simulink model "DigitalControl"  (R2015a)
settings: Solver=ode45  StartTime=0.0  StopTime=10.0  MaxStep=0.1  RelTol=1e-3
undefined symbols (not defined in the file): deltat, deltat1, fden, fnum, Ka, Kf, Ki, Kq, Tal, Ts, W1, W2
libraries: simulink x1
settings Model: FPTRunName=Active  ModifiedByFormat=The MathWorks Inc.  CovSFcnEnable=off  Creator=The MathWorks Inc.  LastModifiedBy=The MathWorks Inc.
settings ConfigSet: ConfigType=Model
settings SolverCC: Priority=auto
settings DataIOCC: SaveOutput=off  SaveTime=off  SignalLoggingName=DigitalControl
settings OptimizationCC: InlineParamsCompatibleMode=off  ExpressionDepthLimit=2147483647  InitFltsAndDblsToZero=on  ForceBlockIOInitOptimize=off  EvaledLifeSpan=1  SimCompilerOptimization=Off
settings DebuggingCC: SaveWithParameterizedLinksMsg=none  UnderspecifiedInitializationDetection=Classic  MergeDetectMultiDrivingBlocksExec=none  SignalResolutionControl=TryResolveAllWithWarning  SolverPrmCheckMsg=warning  MultiTaskDSMMsg=warning  MultiTaskCondExecSysMsg=none  FcnCallInpInsideContextMsg=UseLocalSettings  AllowSymbolicDim=off  StateNameClashWarn=warning  SFMismatchInSimAndRtwBecauseOfMissingDataTypeDiag=warning
settings ModelReferenceCC: ModelReferenceMinAlgLoopOccurrences=on
settings RTWCC: EnableTagging=off  RTWCompilerOptimization=Off
settings CodeAppCC: ParameterTuningSideEffectCode=Output function  AllmanStyle=off
settings GRTTargetCC: TargetFcnLib=ansi_tfl_tmw.mat  CombineOutputUpdateFcns=off  EnableShiftOperators=off  PortableWordSizesTransition=off  GenerateErtSFunctionTransition=off  CreateSILPILBlockTransition=None  CodeProfilingSaveOptionsTransition=SummaryOnly  CodeExecutionProfilingTransition=off  CodeProfilingInstrumentationTransition=off  CodeExecutionProfileVariableTransition=executionProfile  GRTInterface=on

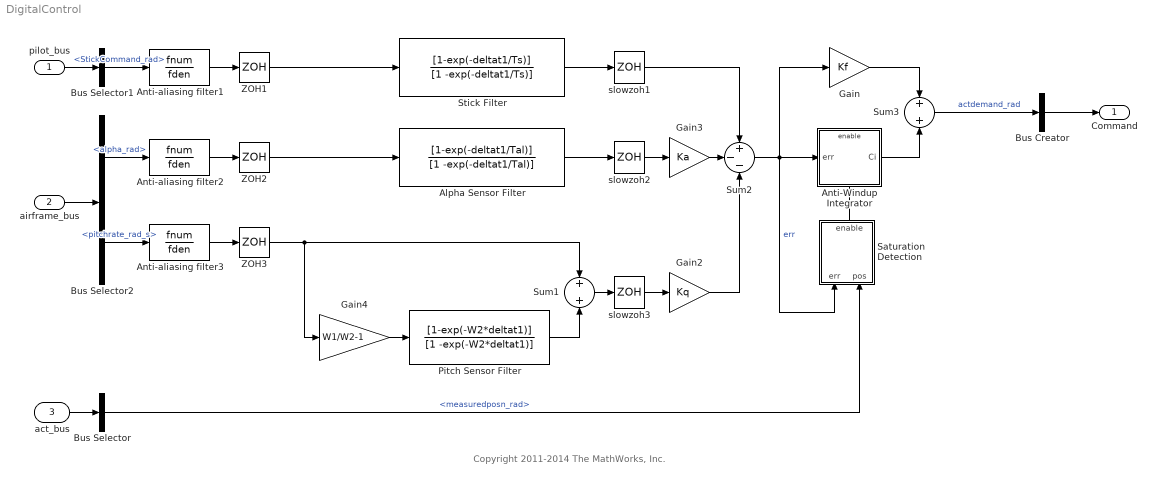
== system DigitalControl ==
  note: Copyright 2011-2014 The MathWorks, Inc.
  pilot_bus : Inport  IOType=none  Commented=off  StatePerturbationForJacobian=1.0e-05  OutDataTypeStr=Bus: PILOT_BUS
  airframe_bus : Inport  IOType=none  Commented=off  StatePerturbationForJacobian=1.0e-05  Port=2  OutDataTypeStr=Bus: AIRFRAME_BUS
  act_bus : Inport  IOType=none  Commented=off  StatePerturbationForJacobian=1.0e-05  Port=3  OutDataTypeStr=Bus: ACT_BUS
  Alpha Sensor Filter : DiscreteTransferFcn  IOType=none  Commented=off  StatePerturbationForJacobian=1.0e-05  Numerator=[1-exp(-deltat1/Tal)]  Denominator=[1 -exp(-deltat1/Tal)]  SampleTime=deltat1
  Anti-Windup Integrator : Subsystem  IOType=none  Commented=off  StatePerturbationForJacobian=1.0e-05  TreatAsAtomicUnit=on
      settings: RTWSystemCode=Inline
  Anti-aliasing filter1 : TransferFcn  IOType=none  Commented=off  StatePerturbationForJacobian=1.0e-05  Numerator=fnum  Denominator=fden
      settings: AttributesFormatString=%<Description>
  Anti-aliasing filter2 : TransferFcn  IOType=none  Commented=off  StatePerturbationForJacobian=1.0e-05  Numerator=fnum  Denominator=fden
      settings: AttributesFormatString=%<Description>
  Anti-aliasing filter3 : TransferFcn  IOType=none  Commented=off  StatePerturbationForJacobian=1.0e-05  Numerator=fnum  Denominator=fden
      settings: AttributesFormatString=%<Description>
  Bus Creator : BusCreator  IOType=none  Commented=off  StatePerturbationForJacobian=1.0e-05  Inputs=1  OutDataTypeStr=Bus: CONTROL_BUS
  Bus Selector : BusSelector  IOType=none  Commented=off  StatePerturbationForJacobian=1.0e-05  OutputSignals=measuredposn_rad
  Bus Selector1 : BusSelector  IOType=none  Commented=off  StatePerturbationForJacobian=1.0e-05  OutputSignals=StickCommand_rad
  Bus Selector2 : BusSelector  IOType=none  Commented=off  StatePerturbationForJacobian=1.0e-05  OutputSignals=alpha_rad,pitchrate_rad_s
  Gain : Gain  IOType=none  Commented=off  StatePerturbationForJacobian=1.0e-05  Gain=Kf  SaturateOnIntegerOverflow=on  OutDataTypeStr=Inherit: Same as input  ParamDataTypeStr=Inherit: Same as input
  Gain2 : Gain  IOType=none  Commented=off  StatePerturbationForJacobian=1.0e-05  Gain=Kq  SaturateOnIntegerOverflow=on  OutDataTypeStr=Inherit: Same as input  ParamDataTypeStr=Inherit: Same as input
  Gain3 : Gain  IOType=none  Commented=off  StatePerturbationForJacobian=1.0e-05  Gain=Ka  SaturateOnIntegerOverflow=on  OutDataTypeStr=Inherit: Same as input  ParamDataTypeStr=Inherit: Same as input
  Gain4 : Gain  IOType=none  Commented=off  StatePerturbationForJacobian=1.0e-05  Gain=W1/W2-1  SaturateOnIntegerOverflow=on  OutDataTypeStr=Inherit: Same as input  ParamDataTypeStr=Inherit: Same as input
  Pitch Sensor Filter : DiscreteTransferFcn  IOType=none  Commented=off  StatePerturbationForJacobian=1.0e-05  Numerator=[1-exp(-W2*deltat1)]  Denominator=[1 -exp(-W2*deltat1)]  SampleTime=deltat1
  Saturation Detection : Subsystem  IOType=none  Commented=off  StatePerturbationForJacobian=1.0e-05
  Stick Filter : DiscreteTransferFcn  IOType=none  Commented=off  StatePerturbationForJacobian=1.0e-05  Numerator=[1-exp(-deltat1/Ts)]  Denominator=[1 -exp(-deltat1/Ts)]  SampleTime=deltat1
  Sum1 : Sum  IOType=none  Commented=off  StatePerturbationForJacobian=1.0e-05  Inputs=2  SaturateOnIntegerOverflow=on  InputSameDT=on  OutDataTypeStr=Inherit: Same as first input
  Sum2 : Sum  IOType=none  Commented=off  StatePerturbationForJacobian=1.0e-05  Inputs=+--  SaturateOnIntegerOverflow=on  InputSameDT=on  OutDataTypeStr=Inherit: Same as first input
  Sum3 : Sum  IOType=none  Commented=off  StatePerturbationForJacobian=1.0e-05  Inputs=2  SaturateOnIntegerOverflow=on  InputSameDT=on  OutDataTypeStr=Inherit: Same as first input
  ZOH1 : ZeroOrderHold  IOType=none  Commented=off  StatePerturbationForJacobian=1.0e-05  SampleTime=deltat1
  ZOH2 : ZeroOrderHold  IOType=none  Commented=off  StatePerturbationForJacobian=1.0e-05  SampleTime=deltat1
  ZOH3 : ZeroOrderHold  IOType=none  Commented=off  StatePerturbationForJacobian=1.0e-05  SampleTime=deltat1
  slowzoh1 : ZeroOrderHold  IOType=none  Commented=off  StatePerturbationForJacobian=1.0e-05  SampleTime=deltat
  slowzoh2 : ZeroOrderHold  IOType=none  Commented=off  StatePerturbationForJacobian=1.0e-05  SampleTime=deltat
  slowzoh3 : ZeroOrderHold  IOType=none  Commented=off  StatePerturbationForJacobian=1.0e-05  SampleTime=deltat
  Command : Outport  IOType=none  Commented=off  StatePerturbationForJacobian=1.0e-05  OutDataTypeStr=Bus: CONTROL_BUS
  wires:
  pilot_bus/1 -> Bus Selector1/1
  act_bus/1 -> Bus Selector/1
  airframe_bus/1 -> Bus Selector2/1
  Bus Creator/1 -> Command/1
  Bus Selector/1 -> Saturation Detection/2(pos)  "<measuredposn_rad>"
  Saturation Detection/1(enable) -> Anti-Windup Integrator/Enable
  ZOH3/1 -> Sum1/1, Gain4/1
  ZOH2/1 -> Alpha Sensor Filter/1
  Anti-aliasing filter3/1 -> ZOH3/1
  Anti-aliasing filter2/1 -> ZOH2/1
  Anti-aliasing filter1/1 -> ZOH1/1
  ZOH1/1 -> Stick Filter/1
  Bus Selector1/1 -> Anti-aliasing filter1/1  "<StickCommand_rad>"
  slowzoh3/1 -> Gain2/1
  Gain4/1 -> Pitch Sensor Filter/1
  Pitch Sensor Filter/1 -> Sum1/2
  Sum1/1 -> slowzoh3/1
  Bus Selector2/2 -> Anti-aliasing filter3/1  "<pitchrate_rad_s>"
  Gain2/1 -> Sum2/3
  Anti-Windup Integrator/1(Ci) -> Sum3/2
  Gain/1 -> Sum3/1
  Gain3/1 -> Sum2/2
  slowzoh2/1 -> Gain3/1
  Alpha Sensor Filter/1 -> slowzoh2/1
  slowzoh1/1 -> Sum2/1
  Stick Filter/1 -> slowzoh1/1
  Bus Selector2/1 -> Anti-aliasing filter2/1  "<alpha_rad>"
  Sum2/1 -> Gain/1, Anti-Windup Integrator/1(err), Saturation Detection/1(err)  "err"
  Sum3/1 -> Bus Creator/1  "actdemand_rad"

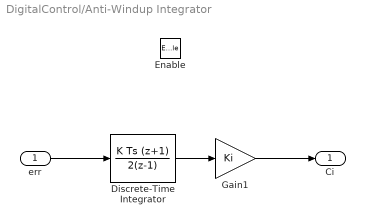
== system DigitalControl/Anti-Windup Integrator ==
  err : Inport  IOType=none  Commented=off  StatePerturbationForJacobian=1.0e-05
  Enable : EnablePort  IOType=none  Commented=off  StatePerturbationForJacobian=1.0e-05
  Discrete-Time Integrator : DiscreteIntegrator  IOType=none  Commented=off  StatePerturbationForJacobian=1.0e-05  IntegratorMethod=Integration: Trapezoidal  SampleTime=deltat
  Gain1 : Gain  IOType=none  Commented=off  StatePerturbationForJacobian=1.0e-05  Gain=Ki  SaturateOnIntegerOverflow=on  OutDataTypeStr=Inherit: Same as input  ParamDataTypeStr=Inherit: Same as input
  Ci : Outport  IOType=none  Commented=off  StatePerturbationForJacobian=1.0e-05  InitialOutput=0
  wires:
  err/1 -> Discrete-Time Integrator/1
  Discrete-Time Integrator/1 -> Gain1/1
  Gain1/1 -> Ci/1

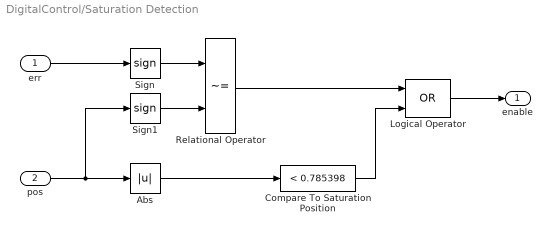
== system DigitalControl/Saturation Detection ==
  err : Inport  IOType=none  Commented=off  StatePerturbationForJacobian=1.0e-05
  pos : Inport  IOType=none  Commented=off  StatePerturbationForJacobian=1.0e-05  Port=2
  Abs : Abs  IOType=none  Commented=off  StatePerturbationForJacobian=1.0e-05  ZeroCross=off
  Compare To Saturation Position : simulink/Logic and Bit Operations/Compare To Constant  IOType=none  Commented=off  StatePerturbationForJacobian=1.0e-05  relop=<  const=0.785398  OutDataTypeStr=boolean  ZeroCross=off
  Logical Operator : Logic  IOType=none  Commented=off  StatePerturbationForJacobian=1.0e-05  Operator=OR  AllPortsSameDT=off  OutDataTypeStr=boolean
  Relational Operator : RelationalOperator  IOType=none  Commented=off  StatePerturbationForJacobian=1.0e-05  Operator=~=  OutDataTypeStr=boolean  ZeroCross=off
  Sign : Signum  IOType=none  Commented=off  StatePerturbationForJacobian=1.0e-05  ZeroCross=off
  Sign1 : Signum  IOType=none  Commented=off  StatePerturbationForJacobian=1.0e-05  ZeroCross=off
  enable : Outport  IOType=none  Commented=off  StatePerturbationForJacobian=1.0e-05
  wires:
  pos/1 -> Sign1/1, Abs/1
  Sign/1 -> Relational Operator/1
  Relational Operator/1 -> Logical Operator/1
  Compare To Saturation Position/1 -> Logical Operator/2
  Sign1/1 -> Relational Operator/2
  Abs/1 -> Compare To Saturation Position/1
  err/1 -> Sign/1
  Logical Operator/1 -> enable/1
